simulink model "EGRVlv_VDSens"  (R2016b)
settings: configuration reference "CodeGenConfigSet" (kept outside this file)
values from neighbouring files (symbols this model uses):
  EGRVlv_facAdapClsStrt_C = Calibration.Parameter    [init_EGRVlv_VDSens.m]
  EGRVlv_facAdapPosCls_C = Calibration.Parameter    [init_EGRVlv_VDSens.m]
  EGRVlv_facPT1_C = Calibration.Parameter    [init_EGRVlv_VDSens.m]
  EGRVlv_facPT1ModVal_C = Calibration.Parameter    [init_EGRVlv_VDSens.m]
  EGRVlv_IKiOfsLrnUp_C = Calibration.Parameter    [init_EGRVlv_VDSens.m]
  EGRVlv_numAdapClsMax_C = Calibration.Parameter    [init_EGRVlv_VDSens.m]
  EGRVlv_numEngTempOfsLrnRls1_C = Calibration.Parameter    [init_EGRVlv_VDSens.m]
  EGRVlv_numEngTempOfsLrnRls2_C = Calibration.Parameter    [init_EGRVlv_VDSens.m]
  EGRVlv_numTempSel_C = Calibration.Parameter    [init_EGRVlv_VDSens.m]
  EGRVlv_rActMax_C = Calibration.Parameter    [init_EGRVlv_VDSens.m]
  EGRVlv_rActMin_C = Calibration.Parameter    [init_EGRVlv_VDSens.m]
  EGRVlv_rActOfs_C = Calibration.Parameter    [init_EGRVlv_VDSens.m]
  EGRVlv_rAdapAgOpnMax_C = Calibration.Parameter    [init_EGRVlv_VDSens.m]
  EGRVlv_rAdapAgOpnMin_C = Calibration.Parameter    [init_EGRVlv_VDSens.m]
  EGRVlv_rAdapDiffPlaus_C = Calibration.Parameter    [init_EGRVlv_VDSens.m]
  EGRVlv_rAdapDiffPlausLgT_C = Calibration.Parameter    [init_EGRVlv_VDSens.m]
  EGRVlv_rAdapDiffPlausShT_C = Calibration.Parameter    [init_EGRVlv_VDSens.m]
  EGRVlv_rAdapIniOpn0_C = Calibration.Parameter    [init_EGRVlv_VDSens.m]
  EGRVlv_rAdapIniOpn_C = Calibration.Parameter    [init_EGRVlv_VDSens.m]
  EGRVlv_rAdapOpnBnd_C = Calibration.Parameter    [init_EGRVlv_VDSens.m]
  EGRVlv_rCmpNewCtlUn_C = Calibration.Parameter    [init_EGRVlv_VDSens.m]
  EGRVlv_RmpSlpNeg_C = Calibration.Parameter    [init_EGRVlv_VDSens.m]
  EGRVlv_RmpSlpPos_C = Calibration.Parameter    [init_EGRVlv_VDSens.m]
  EGRVlv_rOfsLrnDwn_C = Calibration.Parameter    [init_EGRVlv_VDSens.m]
  EGRVlv_rOfsLrnRmpDwnCls_C = Calibration.Parameter    [init_EGRVlv_VDSens.m]
  EGRVlv_rOfsLrnRmpUpFst_C = Calibration.Parameter    [init_EGRVlv_VDSens.m]
  EGRVlv_rOfsLrnVlvMax_C = Calibration.Parameter    [init_EGRVlv_VDSens.m]
  EGRVlv_rOfsLrnVlvMin_C = Calibration.Parameter    [init_EGRVlv_VDSens.m]
  EGRVlv_rOfsMax_C = Calibration.Parameter    [init_EGRVlv_VDSens.m]
  EGRVlv_rOfsMin_C = Calibration.Parameter    [init_EGRVlv_VDSens.m]
  EGRVlv_rPullDwnThres_C = Calibration.Parameter    [init_EGRVlv_VDSens.m]
  EGRVlv_rRmpDwnCls_C = Calibration.Parameter    [init_EGRVlv_VDSens.m]
  EGRVlv_rRmpUpFst_C = Calibration.Parameter    [init_EGRVlv_VDSens.m]
  EGRVlv_rSensVlvThres_C = Calibration.Parameter    [init_EGRVlv_VDSens.m]
  EGRVlv_rTmpOfsLrnMax_C = Calibration.Parameter    [init_EGRVlv_VDSens.m]
  EGRVlv_rTmpOfsLrnMin_C = Calibration.Parameter    [init_EGRVlv_VDSens.m]
  EGRVlv_rTransStgDfl_C = Calibration.Parameter    [init_EGRVlv_VDSens.m]
  EGRVlv_stNewVlvTrg_C = Calibration.Parameter    [init_EGRVlv_VDSens.m]
  EGRVlv_stOfsEngCond_C = Calibration.Parameter    [init_EGRVlv_VDSens.m]
  EGRVlv_stOfsLrnEnb_C = Calibration.Parameter    [init_EGRVlv_VDSens.m]
  EGRVlv_stOfsLrnTrg_C = Calibration.Parameter    [init_EGRVlv_VDSens.m]
  EGRVlv_swtActOfs_C = Calibration.Parameter    [init_EGRVlv_VDSens.m]
  EGRVlv_swtOfsLrnActv_C = Calibration.Parameter    [init_EGRVlv_VDSens.m]
  EGRVlv_swtSensPrs_C = Calibration.Parameter    [init_EGRVlv_VDSens.m]
  EGRVlv_tEngFldThresOfsLrnRls1_C = Calibration.Parameter    [init_EGRVlv_VDSens.m]
  EGRVlv_tEngFldThresOfsLrnRls2_C = Calibration.Parameter    [init_EGRVlv_VDSens.m]
  EGRVlv_tEngMax_C = Calibration.Parameter    [init_EGRVlv_VDSens.m]
  EGRVlv_tEngMin_C = Calibration.Parameter    [init_EGRVlv_VDSens.m]
  EGRVlv_tiAdapJamVlv_C = Calibration.Parameter    [init_EGRVlv_VDSens.m]
  EGRVlv_tiAdapWaitSensAcq_C = Calibration.Parameter    [init_EGRVlv_VDSens.m]
  EGRVlv_tiClsJamVlv_C = Calibration.Parameter    [init_EGRVlv_VDSens.m]
  EGRVlv_tiStable_C = Calibration.Parameter    [init_EGRVlv_VDSens.m]
  EGRVlv_uBattMax_C = Calibration.Parameter    [init_EGRVlv_VDSens.m]
  EGRVlv_uBattMin_C = Calibration.Parameter    [init_EGRVlv_VDSens.m]
  PRC_ZERO = fi(0,Prc_100_rate)    [init_EGRVlv_VDSens.m]
  SigTst_rEGRVlv_C = Calibration.Parameter    [init_EGRVlv_VDSens.m]
  SigTst_swtEGRVlv_C = Calibration.Parameter    [init_EGRVlv_VDSens.m]
undefined symbols (not defined in the file or in its folder): CEngDst_switch_conv, EGRVlv_VDSens_DT, EngState_conv, SubSysExeState_conv, Switch_conv
libraries: simulink x22, CXLib x18
(part 2 of 2)

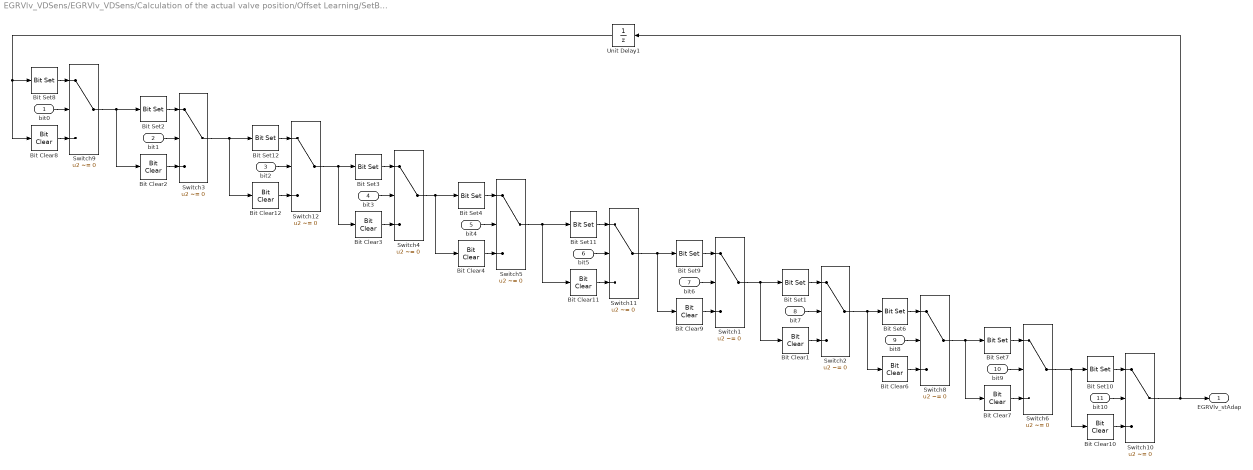
== system EGRVlv_VDSens/EGRVlv_VDSens/Calculation of the actual valve position/Offset Learning/SetBit ==
  bit0 : Inport
  bit1 : Inport  Port=2
  bit2 : Inport  Port=3
  bit3 : Inport  Port=4
  bit4 : Inport  Port=5
  bit5 : Inport  Port=6
  bit6 : Inport  Port=7
  bit7 : Inport  Port=8
  bit8 : Inport  Port=9
  bit9 : Inport  Port=10
  bit10 : Inport  Port=11
  Bit Clear1 : simulink/Logic and Bit Operations/Bit Clear  iBit=7
  Bit Clear10 : simulink/Logic and Bit Operations/Bit Clear  iBit=10
  Bit Clear11 : simulink/Logic and Bit Operations/Bit Clear  iBit=5
  Bit Clear12 : simulink/Logic and Bit Operations/Bit Clear  iBit=2
  Bit Clear2 : simulink/Logic and Bit Operations/Bit Clear  iBit=1
  Bit Clear3 : simulink/Logic and Bit Operations/Bit Clear  iBit=3
  Bit Clear4 : simulink/Logic and Bit Operations/Bit Clear  iBit=4
  Bit Clear6 : simulink/Logic and Bit Operations/Bit Clear  iBit=8
  Bit Clear7 : simulink/Logic and Bit Operations/Bit Clear  iBit=9
  Bit Clear8 : simulink/Logic and Bit Operations/Bit Clear  iBit=0
  Bit Clear9 : simulink/Logic and Bit Operations/Bit Clear  iBit=6
  Bit Set1 : simulink/Logic and Bit Operations/Bit Set  iBit=7
  Bit Set10 : simulink/Logic and Bit Operations/Bit Set  iBit=10
  Bit Set11 : simulink/Logic and Bit Operations/Bit Set  iBit=5
  Bit Set12 : simulink/Logic and Bit Operations/Bit Set  iBit=2
  Bit Set2 : simulink/Logic and Bit Operations/Bit Set  iBit=1
  Bit Set3 : simulink/Logic and Bit Operations/Bit Set  iBit=3
  Bit Set4 : simulink/Logic and Bit Operations/Bit Set  iBit=4
  Bit Set6 : simulink/Logic and Bit Operations/Bit Set  iBit=8
  Bit Set7 : simulink/Logic and Bit Operations/Bit Set  iBit=9
  Bit Set8 : simulink/Logic and Bit Operations/Bit Set  iBit=0
  Bit Set9 : simulink/Logic and Bit Operations/Bit Set  iBit=6
  Switch{1..6,8..12} (11 alike) : Switch  Criteria=u2 ~= 0  OutDataTypeStr=Inherit: Inherit via back propagation  SaturateOnIntegerOverflow=on  InputSameDT=on
  Unit Delay1 : UnitDelay  SampleTime=-1
      settings: AttributesFormatString=InitialValue=%<InitialCondition>
  EGRVlv_stAdap : Outport
  wires:
  bit6/1 -> Switch1/2
  Bit Clear9/1 -> Switch1/3
  bit7/1 -> Switch2/2
  Bit Set9/1 -> Switch1/1
  Switch10/1 -> EGRVlv_stAdap/1, Unit Delay1/1
  Bit Set1/1 -> Switch2/1
  Switch1/1 -> Bit Clear1/1, Bit Set1/1
  Bit Clear1/1 -> Switch2/3
  Bit Clear2/1 -> Switch3/3
  Bit Set2/1 -> Switch3/1
  Bit Clear3/1 -> Switch4/3
  Bit Set3/1 -> Switch4/1
  Unit Delay1/1 -> Bit Clear8/1, Bit Set8/1
  Bit Clear4/1 -> Switch5/3
  Bit Set4/1 -> Switch5/1
  Switch4/1 -> Bit Set4/1, Bit Clear4/1
  bit9/1 -> Switch6/2
  Bit Clear7/1 -> Switch6/3
  Bit Set7/1 -> Switch6/1
  bit8/1 -> Switch8/2
  Bit Clear6/1 -> Switch8/3
  Bit Set6/1 -> Switch8/1
  Switch8/1 -> Bit Set7/1, Bit Clear7/1
  Switch2/1 -> Bit Set6/1, Bit Clear6/1
  Bit Clear8/1 -> Switch9/3
  Bit Set8/1 -> Switch9/1
  Switch9/1 -> Bit Set2/1, Bit Clear2/1
  bit10/1 -> Switch10/2
  Bit Set10/1 -> Switch10/1
  Bit Clear10/1 -> Switch10/3
  Switch6/1 -> Bit Clear10/1, Bit Set10/1
  Bit Clear11/1 -> Switch11/3
  Bit Set11/1 -> Switch11/1
  Switch5/1 -> Bit Clear11/1, Bit Set11/1
  Switch11/1 -> Bit Clear9/1, Bit Set9/1
  bit0/1 -> Switch9/2
  bit1/1 -> Switch3/2
  bit3/1 -> Switch4/2
  bit4/1 -> Switch5/2
  bit5/1 -> Switch11/2
  Bit Clear12/1 -> Switch12/3
  Bit Set12/1 -> Switch12/1
  bit2/1 -> Switch12/2
  Switch12/1 -> Bit Clear3/1, Bit Set3/1
  Switch3/1 -> Bit Clear12/1, Bit Set12/1

== system EGRVlv_VDSens/EGRVlv_VDSens/Calculation of the actual valve position/Offset Learning/State INIT ==
  function : TriggerPort  TriggerType=function-call  VariantControl=Variant
  Constant{,1..3} (4 alike) : Constant  Value=0  OutDataTypeStr=Prc_100_rate
  Constant4 : Constant  Value=0  OutDataTypeStr=Counter_num
  EGRVlv_rAdapLrn_mp : Outport  Tag=%  InitialOutput=0
  EGRVlv_rPosLrnMax_mp : Outport  Tag=%  Port=2
  EGRVlv_rPosLrnMin_mp : Outport  Tag=%  Port=3
  EGRVlv_rAdapPosAvg_mp : Outport  Tag=%  Port=4
  EGRVlv_ctAdapCls_mp : Outport  Port=5
  wires:
  Constant/1 -> EGRVlv_rAdapLrn_mp/1
  Constant1/1 -> EGRVlv_rPosLrnMax_mp/1
  Constant3/1 -> EGRVlv_rAdapPosAvg_mp/1
  Constant2/1 -> EGRVlv_rPosLrnMin_mp/1
  Constant4/1 -> EGRVlv_ctAdapCls_mp/1

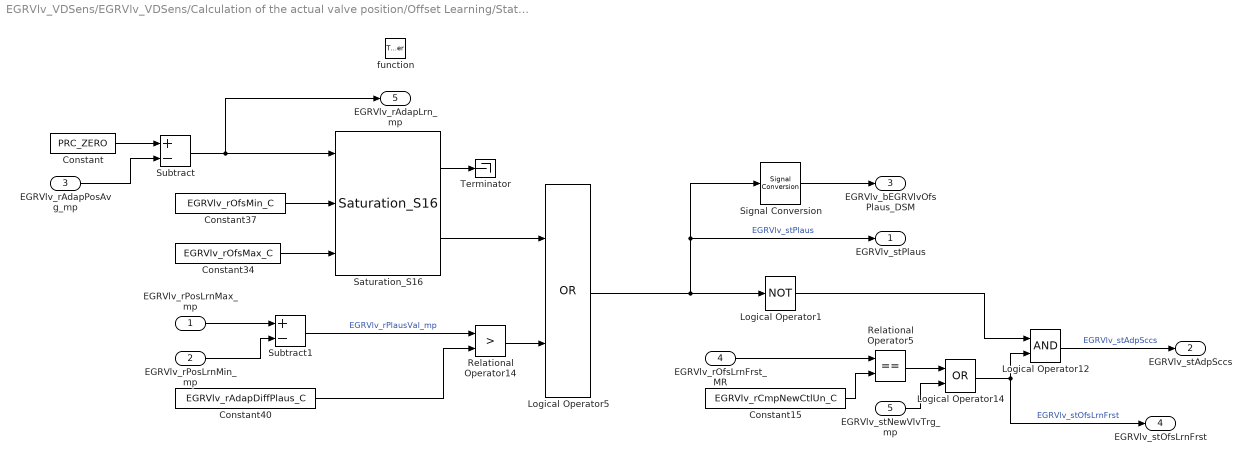
== system EGRVlv_VDSens/EGRVlv_VDSens/Calculation of the actual valve position/Offset Learning/State PLAUSIBLE ==
  EGRVlv_rPosLrnMax_mp : Inport  Tag=%
  EGRVlv_rPosLrnMin_mp : Inport  Tag=%  Port=2
  EGRVlv_rAdapPosAvg_mp : Inport  Tag=%  Port=3
  EGRVlv_rOfsLrnFrst_MR : Inport  Tag=%  Port=4
  EGRVlv_stNewVlvTrg_mp : Inport  Tag=%  Port=5
  function : TriggerPort  TriggerType=function-call  VariantControl=Variant
  Constant : Constant  Value=PRC_ZERO
  Constant15 : Constant  Value=EGRVlv_rCmpNewCtlUn_C  SampleTime=-1
  Constant34 : Constant  Value=EGRVlv_rOfsMax_C  SampleTime=-1
  Constant37 : Constant  Value=EGRVlv_rOfsMin_C  SampleTime=-1
  Constant40 : Constant  Value=EGRVlv_rAdapDiffPlaus_C  SampleTime=-1
  Logical Operator1 : Logic  Operator=NOT  AllPortsSameDT=off  OutDataTypeStr=boolean
  Logical Operator12 : Logic  AllPortsSameDT=off  OutDataTypeStr=boolean
  Logical Operator14 : Logic  Operator=OR  AllPortsSameDT=off  OutDataTypeStr=boolean
  Logical Operator5 : Logic  Operator=OR  AllPortsSameDT=off  OutDataTypeStr=boolean
  Relational Operator14 : RelationalOperator  Operator=>  OutDataTypeStr=boolean  RndMeth=Simplest
  Relational Operator5 : RelationalOperator  Operator===  OutDataTypeStr=boolean  RndMeth=Simplest
  Saturation_S16 : CXLib/Saturation_S16
  Signal Conversion : SignalConversion  OverrideOpt=off
  Subtract : Sum  Inputs=+-  OutDataTypeStr=Inherit: Inherit via back propagation  SaturateOnIntegerOverflow=on  InputSameDT=on
  Subtract1 : Sum  Inputs=+-  SaturateOnIntegerOverflow=on
  Terminator : Terminator
  EGRVlv_stPlaus : Outport  Tag=%
  EGRVlv_stAdpSccs : Outport  Tag=%  Port=2
  EGRVlv_bEGRVlvOfsPlaus_DSM : Outport  Tag=%  Port=3
  EGRVlv_stOfsLrnFrst : Outport  Port=4
  EGRVlv_rAdapLrn_mp : Outport  Tag=%  Port=5  InitialOutput=0
  wires:
  Logical Operator5/1 -> EGRVlv_stPlaus/1, Signal Conversion/1, Logical Operator1/1  "EGRVlv_stPlaus"
  Saturation_S16/2 -> Logical Operator5/1
  Relational Operator14/1 -> Logical Operator5/2
  Subtract1/1 -> Relational Operator14/1  "EGRVlv_rPlausVal_mp"
  Constant40/1 -> Relational Operator14/2
  Constant37/1 -> Saturation_S16/2
  Constant34/1 -> Saturation_S16/3
  Subtract/1 -> Saturation_S16/1, EGRVlv_rAdapLrn_mp/1
  EGRVlv_rPosLrnMax_mp/1 -> Subtract1/1
  EGRVlv_rPosLrnMin_mp/1 -> Subtract1/2
  Signal Conversion/1 -> EGRVlv_bEGRVlvOfsPlaus_DSM/1
  Constant/1 -> Subtract/1
  Logical Operator1/1 -> Logical Operator12/1
  EGRVlv_rOfsLrnFrst_MR/1 -> Relational Operator5/1
  Constant15/1 -> Relational Operator5/2
  Relational Operator5/1 -> Logical Operator14/1
  EGRVlv_stNewVlvTrg_mp/1 -> Logical Operator14/2
  Logical Operator14/1 -> EGRVlv_stOfsLrnFrst/1, Logical Operator12/2  "EGRVlv_stOfsLrnFrst"
  Logical Operator12/1 -> EGRVlv_stAdpSccs/1  "EGRVlv_stAdpSccs"
  EGRVlv_rAdapPosAvg_mp/1 -> Subtract/2
  Saturation_S16/1 -> Terminator/1

== system EGRVlv_VDSens/EGRVlv_VDSens/Calculation of the actual valve position/Offset Learning/State machine for the offset learning for EGR valve/simfcn ==
  EGRVlv_rOfsLrnVlv : Inport  Tag=%
  EGRVlv_rActUnCor : Inport  Port=2  OutDataTypeStr=Prc_100_rate
  EGRVlv_rOfsLrnLst_MR : Inport  Port=3  OutDataTypeStr=Prc_100_rate
  f : TriggerPort  TriggerType=function-call  VariantControl=Variant
      settings: CopyFcn=Stateflow.SLINSF.SimulinkMan.removeBlockPreDeleteFcn  PreDeleteFcn=Stateflow.SLINSF.SimulinkMan.unsafePredeleteFcn
  Add1 : Sum  OutDataTypeStr=Prc_100_rate  SaturateOnIntegerOverflow=on
  Constant10 : Constant  OutDataTypeStr=Prc_100_rate
  Constant11 : Constant  Value=EGRVlv_rAdapOpnBnd_C
  Constant13 : Constant  Value=EGRVlv_rAdapAgOpnMax_C
  Constant7 : Constant  Value=EGRVlv_IKiOfsLrnUp_C
  Integral : Subsystem
  Relational Operator2 : RelationalOperator  OutDataTypeStr=boolean  RndMeth=Simplest
  Switch : Switch  Criteria=u2 ~= 0
  EGRVlv_rOfsLrnVlvUnLim : Outport
  wires:
  Constant10/1 -> Integral/1(Dvt)
  Add1/1 -> Relational Operator2/1
  Constant13/1 -> Relational Operator2/2
  EGRVlv_rActUnCor/1 -> Add1/1
  EGRVlv_rOfsLrnLst_MR/1 -> Add1/2
  Relational Operator2/1 -> Switch/2
  Constant11/1 -> Switch/1
  Switch/1 -> EGRVlv_rOfsLrnVlvUnLim/1
  Integral/1(Out) -> Switch/3
  EGRVlv_rOfsLrnVlv/1 -> Integral/3(InitVal)
  Constant7/1 -> Integral/2(Ki)

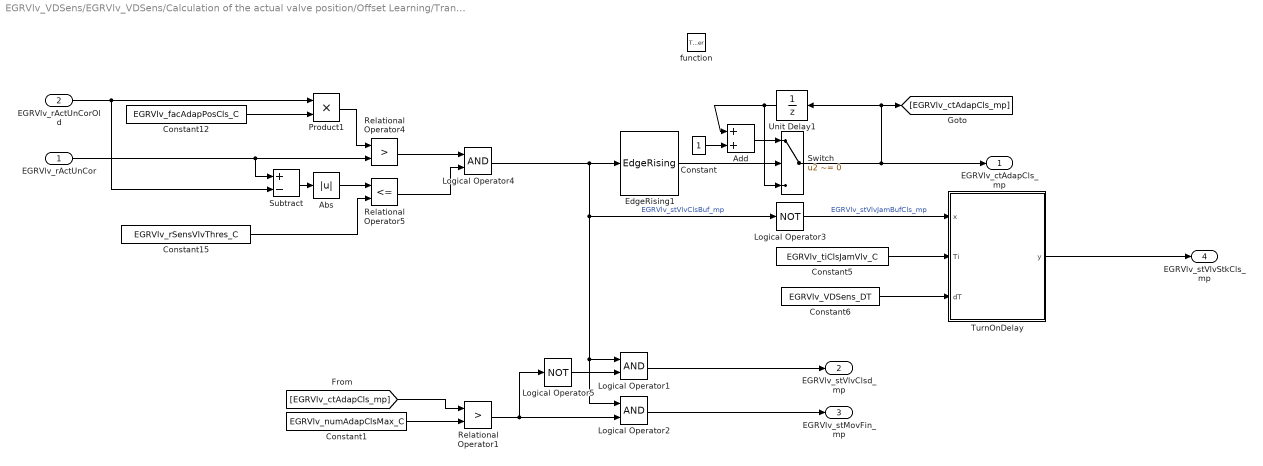
== system EGRVlv_VDSens/EGRVlv_VDSens/Calculation of the actual valve position/Offset Learning/Transition conditions from state CLOSE ==
  EGRVlv_rActUnCor : Inport
  EGRVlv_rActUnCorOld : Inport  Port=2
  function : TriggerPort  TriggerType=function-call  VariantControl=Variant  StatesWhenEnabling=reset
  Abs : Abs
  Add : Sum  SaturateOnIntegerOverflow=on
  Constant : Constant  OutDataTypeStr=Counter_num
  Constant1 : Constant  Value=EGRVlv_numAdapClsMax_C
  Constant12 : Constant  Value=EGRVlv_facAdapPosCls_C
  Constant15 : Constant  Value=EGRVlv_rSensVlvThres_C
  Constant5 : Constant  Value=EGRVlv_tiClsJamVlv_C
  Constant6 : Constant  Value=EGRVlv_VDSens_DT
  EdgeRising1 : CXLib/EdgeRising
  Logical Operator1 : Logic  AllPortsSameDT=off  OutDataTypeStr=boolean
  Logical Operator2 : Logic  AllPortsSameDT=off  OutDataTypeStr=boolean
  Logical Operator3 : Logic  Operator=NOT  AllPortsSameDT=off  OutDataTypeStr=boolean
  Logical Operator4 : Logic  AllPortsSameDT=off  OutDataTypeStr=boolean
  Logical Operator5 : Logic  Operator=NOT  AllPortsSameDT=off  OutDataTypeStr=boolean
  Product1 : Product  OutDataTypeStr=Prc_100_rate  SaturateOnIntegerOverflow=on
  Relational Operator1 : RelationalOperator  Operator=>  OutDataTypeStr=boolean  RndMeth=Simplest
  Relational Operator4 : RelationalOperator  Operator=>  OutDataTypeStr=boolean  RndMeth=Simplest
  Relational Operator5 : RelationalOperator  Operator=<=  OutDataTypeStr=boolean  RndMeth=Simplest
  Subtract : Sum  Inputs=+-  SaturateOnIntegerOverflow=on
  Switch : Switch  Criteria=u2 ~= 0
  TurnOnDelay : Subsystem
  Unit Delay1 : UnitDelay  SampleTime=-1
      settings: AttributesFormatString=InitialValue=%<InitialCondition>
  EGRVlv_ctAdapCls_mp : Outport
  EGRVlv_stVlvClsd_mp : Outport  Port=2  InitialOutput=0
  EGRVlv_stMovFin_mp : Outport  Port=3  InitialOutput=0
  EGRVlv_stVlvStkCls_mp : Outport  Port=4  InitialOutput=0
  wires:
  Logical Operator4/1 -> EdgeRising1/1, Logical Operator3/1, Logical Operator2/1, Logical Operator1/1  "EGRVlv_stVlvClsBuf_mp"
  Constant5/1 -> TurnOnDelay/2(Ti)
  Constant6/1 -> TurnOnDelay/3(dT)
  Logical Operator3/1 -> TurnOnDelay/1(x)  "EGRVlv_stVlvJamBufCls_mp"
  EGRVlv_rActUnCor/1 -> Subtract/1, Relational Operator4/2
  Constant12/1 -> Product1/2
  Product1/1 -> Relational Operator4/1
  Relational Operator4/1 -> Logical Operator4/1
  EGRVlv_rActUnCorOld/1 -> Subtract/2, Product1/1
  Subtract/1 -> Abs/1
  Abs/1 -> Relational Operator5/1
  Constant15/1 -> Relational Operator5/2
  Relational Operator5/1 -> Logical Operator4/2
  Constant/1 -> Add/2
  Add/1 -> Switch/1
  Unit Delay1/1 -> Switch/3, Add/1
  Switch/1 -> EGRVlv_ctAdapCls_mp/1, Unit Delay1/1, [EGRVlv_ctAdapCls_mp]
  Logical Operator1/1 -> EGRVlv_stVlvClsd_mp/1
  Logical Operator2/1 -> EGRVlv_stMovFin_mp/1
  Logical Operator5/1 -> Logical Operator1/2
  Constant1/1 -> Relational Operator1/2
  Relational Operator1/1 -> Logical Operator5/1, Logical Operator2/2
  [EGRVlv_ctAdapCls_mp] -> Relational Operator1/1
  EdgeRising1/1 -> Switch/2
  TurnOnDelay/1(y) -> EGRVlv_stVlvStkCls_mp/1

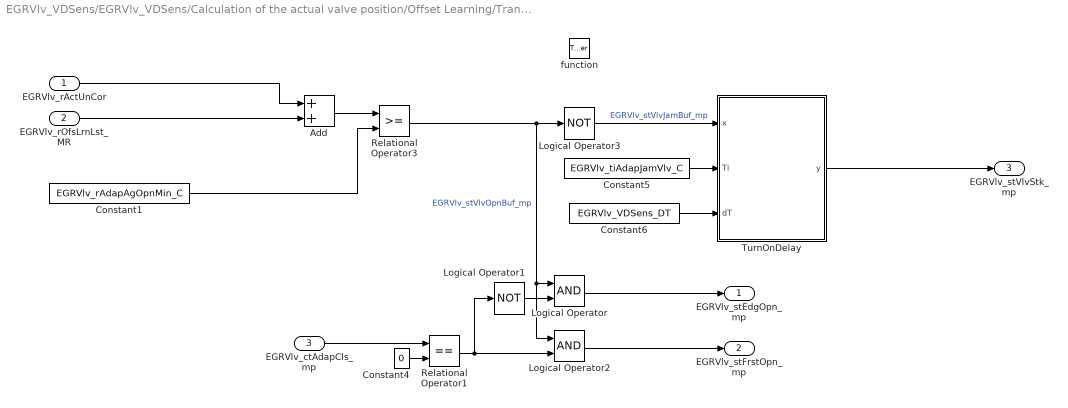
== system EGRVlv_VDSens/EGRVlv_VDSens/Calculation of the actual valve position/Offset Learning/Transition conditions from state OPEN ==
  EGRVlv_rActUnCor : Inport
  EGRVlv_rOfsLrnLst_MR : Inport  Port=2
  EGRVlv_ctAdapCls_mp : Inport  Tag=%  Port=3
  function : TriggerPort  TriggerType=function-call  VariantControl=Variant
  Add : Sum  SaturateOnIntegerOverflow=on
  Constant1 : Constant  Value=EGRVlv_rAdapAgOpnMin_C
  Constant4 : Constant  Value=0  OutDataTypeStr=Inherit: Inherit via back propagation
  Constant5 : Constant  Value=EGRVlv_tiAdapJamVlv_C
  Constant6 : Constant  Value=EGRVlv_VDSens_DT
  Logical Operator : Logic  AllPortsSameDT=off  OutDataTypeStr=boolean
  Logical Operator1 : Logic  Operator=NOT  AllPortsSameDT=off  OutDataTypeStr=boolean
  Logical Operator2 : Logic  AllPortsSameDT=off  OutDataTypeStr=boolean
  Logical Operator3 : Logic  Operator=NOT  AllPortsSameDT=off  OutDataTypeStr=boolean
  Relational Operator1 : RelationalOperator  Operator===  OutDataTypeStr=boolean  RndMeth=Simplest  InputSameDT=on
  Relational Operator3 : RelationalOperator  OutDataTypeStr=boolean  RndMeth=Simplest
  TurnOnDelay : Subsystem
  EGRVlv_stEdgOpn_mp : Outport  InitialOutput=0
  EGRVlv_stFrstOpn_mp : Outport  Port=2  InitialOutput=0
  EGRVlv_stVlvStk_mp : Outport  Port=3  InitialOutput=0
  wires:
  Add/1 -> Relational Operator3/1
  Constant1/1 -> Relational Operator3/2
  Relational Operator3/1 -> Logical Operator2/1, Logical Operator/1, Logical Operator3/1  "EGRVlv_stVlvOpnBuf_mp"
  EGRVlv_ctAdapCls_mp/1 -> Relational Operator1/1
  Constant4/1 -> Relational Operator1/2
  Logical Operator1/1 -> Logical Operator/2
  Relational Operator1/1 -> Logical Operator1/1, Logical Operator2/2
  Logical Operator/1 -> EGRVlv_stEdgOpn_mp/1
  Logical Operator2/1 -> EGRVlv_stFrstOpn_mp/1
  Constant5/1 -> TurnOnDelay/2(Ti)
  Constant6/1 -> TurnOnDelay/3(dT)
  Logical Operator3/1 -> TurnOnDelay/1(x)  "EGRVlv_stVlvJamBuf_mp"
  EGRVlv_rOfsLrnLst_MR/1 -> Add/2
  EGRVlv_rActUnCor/1 -> Add/1
  TurnOnDelay/1(y) -> EGRVlv_stVlvStk_mp/1

== system EGRVlv_VDSens/EGRVlv_VDSens/Calculation of the actual valve position/Offset Learning/Transition conditions from state Store ==
  EGRVlv_rAdapPos_mp : Inport  Tag=%
  EGRVlv_ctAdapCls_mp : Inport  Tag=%  Port=2
  function : TriggerPort  TriggerType=function-call  VariantControl=Variant
  Add : Sum  SaturateOnIntegerOverflow=on
  Constant1 : Constant  Value=0  OutDataTypeStr=Counter_num  SampleTime=-1
  Divide : Product  Inputs=*/  OutDataTypeStr=Prc_100_rate  SaturateOnIntegerOverflow=on
  Relational Operator1 : RelationalOperator  Operator=~=  OutDataTypeStr=boolean  RndMeth=Simplest
  Relational Operator4 : RelationalOperator  Operator=>  OutDataTypeStr=boolean  RndMeth=Simplest
  Relational Operator5 : RelationalOperator  Operator=<  OutDataTypeStr=boolean  RndMeth=Simplest
  Switch1 : Switch  Criteria=u2 ~= 0  Threshold=CEngDst_switch_conv.OFF  InputSameDT=on
  Switch7 : Switch  Criteria=u2 ~= 0  Threshold=CEngDst_switch_conv.OFF  InputSameDT=on
  Switch8 : Switch  Criteria=u2 ~= 0  Threshold=CEngDst_switch_conv.OFF  InputSameDT=on
  Unit Delay : UnitDelay  InitialCondition=-100  SampleTime=-1
      settings: AttributesFormatString=InitialValue=%<InitialCondition>
  Unit Delay1 : UnitDelay  InitialCondition=100  SampleTime=-1
      settings: AttributesFormatString=InitialValue=%<InitialCondition>
  Unit Delay2 : UnitDelay  SampleTime=-1
      settings: AttributesFormatString=InitialValue=%<InitialCondition>
  EGRVlv_rPosLrnMax_mp : Outport  Tag=%
  EGRVlv_rPosLrnMin_mp : Outport  Tag=%  Port=2
  EGRVlv_rAdapPosAvg_mp : Outport  Tag=%  Port=3
  wires:
  Relational Operator1/1 -> Switch1/2
  Unit Delay/1 -> Relational Operator4/2, Switch7/3
  Unit Delay1/1 -> Switch8/3, Relational Operator5/2
  Switch8/1 -> EGRVlv_rPosLrnMin_mp/1, Unit Delay1/1
  Relational Operator5/1 -> Switch8/2
  Relational Operator4/1 -> Switch7/2
  Constant1/1 -> Relational Operator1/2
  Divide/1 -> Switch1/1
  Unit Delay2/1 -> Add/1
  EGRVlv_ctAdapCls_mp/1 -> Relational Operator1/1, Divide/2
  Switch7/1 -> EGRVlv_rPosLrnMax_mp/1, Unit Delay/1
  EGRVlv_rAdapPos_mp/1 -> Switch1/3, Switch8/1, Relational Operator5/1, Relational Operator4/1, Switch7/1, Add/2
  Switch1/1 -> EGRVlv_rAdapPosAvg_mp/1
  Add/1 -> Divide/1, Unit Delay2/1

== system EGRVlv_VDSens/EGRVlv_VDSens/Calculation of the actual valve position/Offset Learning/State machine for the offset learning for EGR valve/simfcn/Integral ==
  note: Outport
      | should inherit data type from back
  Dvt : Inport
  Ki : Inport  Port=2
  InitVal : Inport  Port=3
  Data Type Duplicate : DataTypeDuplicate
  Product3 : Product  OutDataTypeStr=Inherit: Inherit via back propagation  SaturateOnIntegerOverflow=on
  Sum : Sum  OutDataTypeStr=Inherit: Inherit via back propagation  SaturateOnIntegerOverflow=on  InputSameDT=on
  Out : Outport
  wires:
  Dvt/1 -> Product3/1
  Sum/1 -> Out/1, Data Type Duplicate/1
  InitVal/1 -> Sum/1, Data Type Duplicate/2
  Product3/1 -> Sum/2
  Ki/1 -> Product3/2

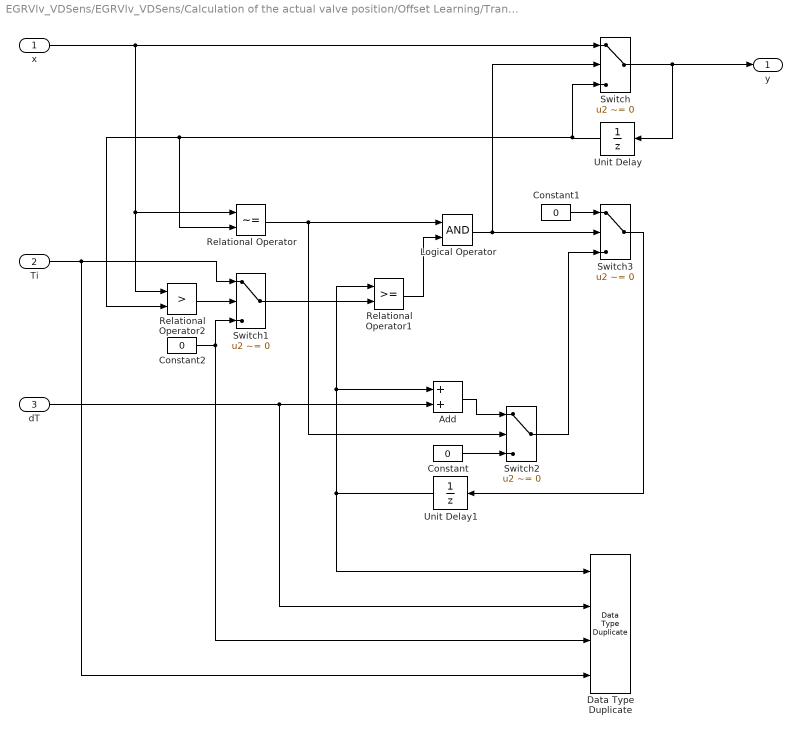
== system EGRVlv_VDSens/EGRVlv_VDSens/Calculation of the actual valve position/Offset Learning/Transition conditions from state CLOSE/TurnOnDelay ==
  x : Inport
  Ti : Inport  Port=2
  dT : Inport  Port=3
  Add : Sum  SaturateOnIntegerOverflow=on
  Constant : Constant  Value=0  OutDataTypeStr=Inherit: Inherit via back propagation
  Constant1 : Constant  Value=0  OutDataTypeStr=Inherit: Inherit via back propagation
  Constant2 : Constant  Value=0  OutDataTypeStr=Inherit: Inherit via back propagation
  Data Type Duplicate : DataTypeDuplicate  NumInputPorts=4
  Logical Operator : Logic  OutDataTypeStr=boolean
  Relational Operator : RelationalOperator  Operator=~=  OutDataTypeStr=boolean  RndMeth=Simplest  InputSameDT=on
  Relational Operator1 : RelationalOperator  OutDataTypeStr=boolean  RndMeth=Simplest  InputSameDT=on
  Relational Operator2 : RelationalOperator  Operator=>  OutDataTypeStr=boolean  RndMeth=Simplest  InputSameDT=on
  Switch{,1..3} (4 alike) : Switch  Criteria=u2 ~= 0  InputSameDT=on
  Unit Delay : UnitDelay  SampleTime=-1
  Unit Delay1 : UnitDelay  SampleTime=-1
  y : Outport
  wires:
  Relational Operator/1 -> Logical Operator/1, Switch2/2
  dT/1 -> Data Type Duplicate/2, Add/2
  Unit Delay1/1 -> Relational Operator1/1, Add/1, Data Type Duplicate/1
  Constant2/1 -> Data Type Duplicate/3, Switch1/3
  x/1 -> Switch/1, Relational Operator2/1, Relational Operator/1
  Switch2/1 -> Switch3/3
  Constant1/1 -> Switch3/1
  Unit Delay/1 -> Relational Operator2/2, Relational Operator/2, Switch/3
  Relational Operator2/1 -> Switch1/2
  Switch3/1 -> Unit Delay1/1
  Ti/1 -> Data Type Duplicate/4, Switch1/1
  Constant/1 -> Switch2/3
  Relational Operator1/1 -> Logical Operator/2
  Add/1 -> Switch2/1
  Switch/1 -> y/1, Unit Delay/1
  Switch1/1 -> Relational Operator1/2
  Logical Operator/1 -> Switch/2, Switch3/2

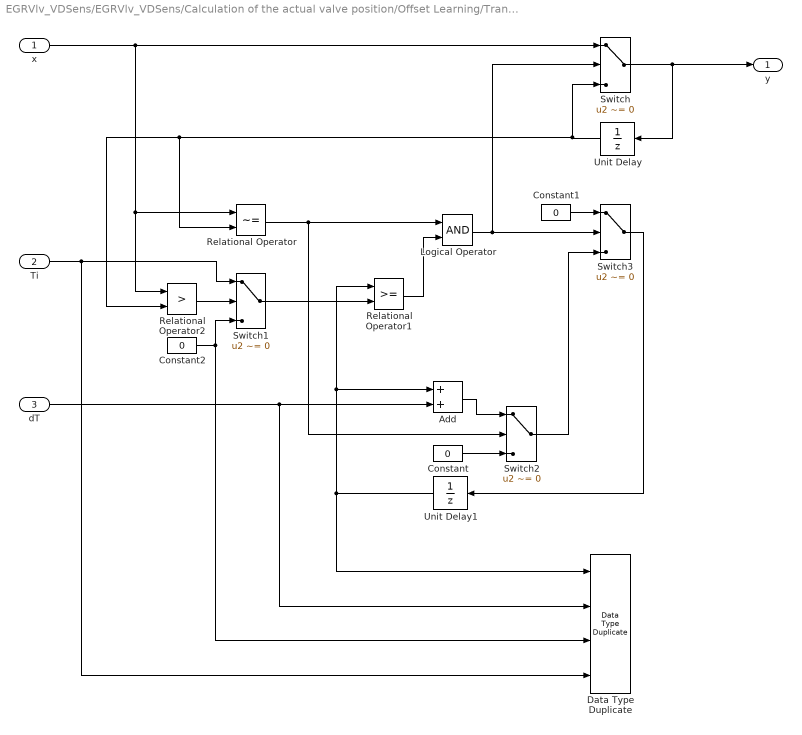
== system EGRVlv_VDSens/EGRVlv_VDSens/Calculation of the actual valve position/Offset Learning/Transition conditions from state OPEN/TurnOnDelay ==
  x : Inport
  Ti : Inport  Port=2
  dT : Inport  Port=3
  Add : Sum  SaturateOnIntegerOverflow=on
  Constant : Constant  Value=0  OutDataTypeStr=Inherit: Inherit via back propagation
  Constant1 : Constant  Value=0  OutDataTypeStr=Inherit: Inherit via back propagation
  Constant2 : Constant  Value=0  OutDataTypeStr=Inherit: Inherit via back propagation
  Data Type Duplicate : DataTypeDuplicate  NumInputPorts=4
  Logical Operator : Logic  OutDataTypeStr=boolean
  Relational Operator : RelationalOperator  Operator=~=  OutDataTypeStr=boolean  RndMeth=Simplest  InputSameDT=on
  Relational Operator1 : RelationalOperator  OutDataTypeStr=boolean  RndMeth=Simplest  InputSameDT=on
  Relational Operator2 : RelationalOperator  Operator=>  OutDataTypeStr=boolean  RndMeth=Simplest  InputSameDT=on
  Switch{,1..3} (4 alike) : Switch  Criteria=u2 ~= 0  InputSameDT=on
  Unit Delay : UnitDelay  SampleTime=-1
  Unit Delay1 : UnitDelay  SampleTime=-1
  y : Outport
  wires:
  Relational Operator/1 -> Logical Operator/1, Switch2/2
  dT/1 -> Data Type Duplicate/2, Add/2
  Unit Delay1/1 -> Relational Operator1/1, Add/1, Data Type Duplicate/1
  Constant2/1 -> Data Type Duplicate/3, Switch1/3
  x/1 -> Switch/1, Relational Operator2/1, Relational Operator/1
  Switch2/1 -> Switch3/3
  Constant1/1 -> Switch3/1
  Unit Delay/1 -> Relational Operator2/2, Relational Operator/2, Switch/3
  Relational Operator2/1 -> Switch1/2
  Switch3/1 -> Unit Delay1/1
  Ti/1 -> Data Type Duplicate/4, Switch1/1
  Constant/1 -> Switch2/3
  Relational Operator1/1 -> Logical Operator/2
  Add/1 -> Switch2/1
  Switch/1 -> y/1, Unit Delay/1
  Switch1/1 -> Relational Operator1/2
  Logical Operator/1 -> Switch/2, Switch3/2

== stateflow chart EGRVlv_VDSens/Calculation of the actual valve position/Offset Learning/State machine for the offset learning for EGR valve ==
  state EGRVlv_rOfsLrnVlvUnLim = simfcn(EGRVlv_rOfsLrnVlv,EGRVlv_rActUnCor,EGRVlv_rOfsLrnLst_MR) [function]
  state EGRVLV_ST_OPN
    entry:
    EGRVlv_stOfsLrn = 2;
    EGRVlv_stAdapVlv_mp = 0;
    Open;
    during:
    Open;
    EGRVlv_rOfsLrnVlvUnLim = simfcn(EGRVlv_rOfsLrnVlv,EGRVlv_rActUnCor,EGRVlv_rOfsLrnLst_MR);
    (default) -> (junction 330)
    (junction 330) -> (junction 331) [order 1] : [EGRVlv_ctAdapCls_mp == 0]
    (junction 330) -> (junction 332) [order 2] : {EGRVlv_rOfsLrnVlvUnLim = EGRVlv_rAdapIniOpn_C;}
    (junction 331) -> (junction 333) : {EGRVlv_rOfsLrnVlvUnLim = EGRVlv_rEGR + EGRVlv_rAdapIniOpn0_C;}
    (junction 333) -> (junction 332)
    (junction 332) -> (junction 334)
  state EGRVLV_ST_CLS
    entry:
    EGRVlv_stOfsLrn = 3;
    EGRVlv_stAdapVlv_mp = 1;
    EGRVlv_rOfsLrnVlvUnLim = EGRVlv_rOfsLrnVlv * EGRVlv_facAdapClsStrt_C;
    Close;
    during:
    Close;
    EGRVlv_rOfsLrnVlvUnLim = EGRVlv_rOfsLrnVlv - EGRVlv_rOfsLrnDwn_C;
  state EGRVLV_ST_INIT
    entry:
    EGRVlv_stOfsLrn = 1;
    EGRVlv_bEGRVlvOfsLrnJamVlv_DSM = 0;
    EGRVlv_stLgTDrft = 0;
    EGRVlv_stShTDrft = 0;
    Init;
  state EGRVLV_ST_RMPDWNCLS
    entry:
    EGRVlv_stOfsLrn = 17;
    EGRVlv_stIntegRmpDwnCls_mp = 0;
    EGRVLV_ST_RMPDWNCLS -> (junction 156) [order 1]
    (junction 156) -> (junction 158) [order 1] : [EGRVlv_rOfsLrnVlvUnLim<=EGRVlv_rRmpDwnCls_C]
    (junction 156) -> (junction 161) [order 2] : {EGRVlv_rOfsLrnVlvUnLim = EGRVlv_rOfsLrnVlv - EGRVlv_rOfsLrnRmpDwnCls_C;}
    (junction 158) -> (junction 160) : {EGRVlv_stIntegRmpDwnCls_mp = 1;}
    (junction 160) -> (junction 161)
    (junction 161) -> (junction 165)
  state EGRVLV_ST_RMPUPFST
    entry:
    EGRVlv_stOfsLrn = 18;
    EGRVlv_stIntegRmpUpFst_mp = 0;
    EGRVLV_ST_RMPUPFST -> (junction 174) [order 1]
    (junction 174) -> (junction 175) [order 1] : [EGRVlv_rOfsLrnVlvUnLim>=EGRVlv_rRmpUpFst_C]
    (junction 174) -> (junction 172) [order 2] : {EGRVlv_rOfsLrnVlvUnLim = EGRVlv_rOfsLrnVlv + EGRVlv_rOfsLrnRmpUpFst_C;}
    (junction 175) -> (junction 169) : {EGRVlv_tiStable_mp+=DT;}
    (junction 169) -> (junction 179) [order 1] : [EGRVlv_tiStable_mp>=EGRVlv_tiStable_C]
    (junction 169) -> (junction 178) [order 2]
    (junction 179) -> (junction 180) : {EGRVlv_stIntegRmpUpFst_mp = 1;}
    (junction 178) -> (junction 172)
    (junction 180) -> (junction 178)
    (junction 172) -> (junction 187)
  state EGRVLV_ST_WAITSENSACQ
    entry:
    EGRVlv_stOfsLrn = 19;
    EGRVlv_stWaitElaps = 0;
    EGRVLV_ST_WAITSENSACQ -> (junction 287) [order 1]
    (junction 287) -> (junction 288) [order 1] : [EGRVlv_tiAdapWaitSensAcq_mp>=EGRVlv_tiAdapWaitSensAcq_C]
    (junction 287) -> (junction 290) [order 2] : {EGRVlv_tiAdapWaitSensAcq_mp+=DT;}
    (junction 288) -> (junction 291) : {EGRVlv_stWaitElaps = 1;
        | EGRVlv_tiAdapWaitSensAcq_mp = 0;}
    (junction 291) -> (junction 290)
    (junction 290) -> (junction 289)
  state EGRVLV_ST_STR
    entry:
    EGRVlv_stOfsLrn = 12;
    EGRVlv_stStr_mp = 0;
    during:
    EGRVlv_rAdapPos_mp = EGRVlv_rActUnCor;
    Store;
    EGRVlv_stStr_mp = 1;
  state EGRVLV_ST_SHOFF
    entry:
    EGRVlv_stOfsLrn = 8;
    EGRVlv_rOfsLrnVlvUnLim = 0;
    EGRVlv_bEGRVlvOfsLrnJamVlv_DSM = 1;
  state EGRVLV_ST_PLAUS
    entry:
    EGRVlv_stOfsLrn = 9;
    Plausible;
    during:
    Plausible;
  state EGRVLV_ST_RMTVAL
    entry:
    EGRVlv_stOfsLrn = 7;
    EGRVlv_rOfsLrnVlvUnLim = 0;
    EGRVlv_stAdapFin = 1;
  state EGRVLV_ST_LGTDRFT
    entry:
    EGRVlv_stOfsLrn = 10;
    EGRVlv_stLgTDrft = 0;
    EGRVlv_bEGRVlvLgTDrft_DSM = 0;
    (default) -> (junction 264)
    EGRVLV_ST_LGTDRFT -> (junction 264) [order 1]
    (junction 264) -> (junction 265) [order 1] : [abs(EGRVlv_rAdapPosAvg_mp-EGRVlv_rOfsLrnFrst_MR)>EGRVlv_rAdapDiffPlausLgT_C]
    (junction 265) -> (junction 268) : {EGRVlv_stLgTDrft = 1;
        | EGRVlv_bEGRVlvLgTDrft_DSM = 1;}
    (junction 264) -> (junction 266) [order 2]
    (junction 268) -> (junction 266)
    (junction 266) -> (junction 267)
  state EGRVLV_ST_SHTDRFT
    entry:
    EGRVlv_stOfsLrn = 11;
    EGRVlv_stShTDrft = 0;
    EGRVlv_bEGRVlvShTDrft_DSM = 0;
    (default) -> (junction 276)
    EGRVLV_ST_SHTDRFT -> (junction 276) [order 1]
    (junction 276) -> (junction 280) [order 1] : [abs(EGRVlv_rAdapPosAvg_mp-EGRVlv_rOfsLrnLst_MR)>EGRVlv_rAdapDiffPlausShT_C]
    (junction 276) -> (junction 281) [order 2]
    (junction 280) -> (junction 275) : {EGRVlv_stShTDrft = 1;
        | EGRVlv_bEGRVlvShTDrft_DSM = 1;}
    (junction 275) -> (junction 281)
    (junction 281) -> (junction 277)
  state EGRVLV_ST_ADAPSCCS
    entry:
    EGRVlv_stOfsLrn = 6;
    EGRVlv_rOfsLrnVlvUnLim = 0;
    EGRVlv_stAdapFin = 1;
    EGRVlv_rOfsLrnLst_MW = EGRVlv_rAdapPosAvg_mp;
    (default) -> (junction 253)
    (junction 253) -> (junction 254) [order 1] : [EGRVlv_stOfsLrnFrst == 1]
    (junction 253) -> (junction 257) [order 2]
    (junction 254) -> (junction 256) : {EGRVlv_rOfsLrnFrst_MW = EGRVlv_rAdapPosAvg_mp;}
    (junction 256) -> (junction 257)
    (junction 257) -> (junction 258)
  (default) -> EGRVLV_ST_INIT : {EGRVlv_rOfsLrnFrst_MW = EGRVlv_rOfsLrnFrst_MR;
      | EGRVlv_rOfsLrnLst_MW = EGRVlv_rOfsLrnLst_MR;}
  EGRVLV_ST_CLS -> EGRVLV_ST_PLAUS [order 2] : [EGRVlv_stMovFin_mp == 1]
  EGRVLV_ST_INIT -> EGRVLV_ST_OPN : [EGRVlv_stTrg_mp == 1]
  EGRVLV_ST_OPN -> EGRVLV_ST_CLS [order 2] : [(EGRVlv_stFrstOpn_mp == 1)||...
      | ((EGRVlv_stEdgOpn_mp == 1)&&...
      | (EGRVlv_swtEGRTyp2 == 1))]
  EGRVLV_ST_CLS -> EGRVLV_ST_SHOFF [order 3] : [EGRVlv_stVlvStkCls_mp == 1]
  EGRVLV_ST_STR -> EGRVLV_ST_CLS [order 2] : [(EGRVlv_stAdapVlv_mp == 0) &&...
      | (EGRVlv_stStr_mp == 1)]
  EGRVLV_ST_CLS -> EGRVLV_ST_RMPDWNCLS [order 1] : [(EGRVlv_stVlvClsd_mp == 1)&&...
      | (EGRVlv_swtEGRTyp2T == 1)]
  EGRVLV_ST_ADAPSCCS -> EGRVLV_ST_INIT
  EGRVLV_ST_RMTVAL -> EGRVLV_ST_INIT
  EGRVLV_ST_OPN -> EGRVLV_ST_SHOFF [order 1] : [EGRVlv_stVlvStk_mp == 1]
  EGRVLV_ST_STR -> EGRVLV_ST_OPN [order 1] : [(EGRVlv_stAdapVlv_mp == 1) &&...
      | (EGRVlv_stStr_mp == 1)]
  EGRVLV_ST_RMPDWNCLS -> EGRVLV_ST_RMPUPFST [order 1] : [(EGRVlv_stIntegRmpDwnCls_mp ==1)&&...
      | ((EGRVlv_swtEGRTyp2T == 1))]
  EGRVLV_ST_RMPUPFST -> EGRVLV_ST_WAITSENSACQ [order 1] : [(EGRVlv_stIntegRmpUpFst_mp ==1)&&...
      | (EGRVlv_swtEGRTyp2T == 1)]
      | {EGRVlv_tiStable_mp =0;}
  EGRVLV_ST_WAITSENSACQ -> EGRVLV_ST_STR [order 1] : [EGRVlv_stWaitElaps == 1]
  EGRVLV_ST_SHOFF -> EGRVLV_ST_RMTVAL
  EGRVLV_ST_PLAUS -> EGRVLV_ST_RMTVAL [order 3] : [EGRVlv_stPlaus ==1]
  EGRVLV_ST_PLAUS -> EGRVLV_ST_ADAPSCCS [order 1] : [EGRVlv_stAdpSccs == 1]
  EGRVLV_ST_PLAUS -> EGRVLV_ST_LGTDRFT [order 2] : [EGRVlv_stPlaus == 0]
  EGRVLV_ST_LGTDRFT -> EGRVLV_ST_RMTVAL [order 2] : [EGRVlv_stLgTDrft ==1]
  EGRVLV_ST_SHTDRFT -> EGRVLV_ST_RMTVAL [order 2] : [EGRVlv_stShTDrft ==1]
  EGRVLV_ST_LGTDRFT -> EGRVLV_ST_SHTDRFT [order 1] : [EGRVlv_stLgTDrft  == 0]
  EGRVLV_ST_SHTDRFT -> EGRVLV_ST_ADAPSCCS [order 1] : [EGRVlv_stShTDrft == 0]
  data: EGRVlv_rOfsLrnVlv function_input; EGRVlv_rOfsLrnVlvUnLim function_output; EGRVlv_rActUnCor function_input Prc_100_rate; EGRVlv_rOfsLrnLst_MR function_input Prc_100_rate; EGRVlv_rOfsLrnVlv input; EGRVlv_rEGR input; EGRVlv_rOfsLrnVlvUnLim output Prc_100_rate; EGRVlv_rAdapIniOpn_C input; EGRVlv_rAdapIniOpn0_C input; EGRVlv_facAdapClsStrt_C input; EGRVlv_rOfsLrnRmpUpFst_C input; EGRVlv_rOfsLrnRmpDwnCls_C input; EGRVlv_ctAdapCls_mp input; EGRVlv_swtEGRTyp2 input; EGRVlv_stTrg_mp input; EGRVlv_swtEGRTyp2T input; EGRVlv_rOfsLrnDwn_C input; EGRVlv_rRmpDwnCls_C input; EGRVlv_rRmpUpFst_C input; EGRVlv_tiStable_C input; EGRVlv_stAdapFin output boolean; EGRVlv_stAdapVlv_mp output boolean; EGRVlv_bEGRVlvOfsLrnJamVlv_DSM output boolean; EGRVlv_stLgTDrft output boolean; EGRVlv_stShTDrft output boolean; EGRVlv_stOfsLrn output State_uint8; EGRVlv_stStr_mp output boolean; EGRVlv_stIntegRmpDwnCls_mp local boolean; EGRVlv_stIntegRmpUpFst_mp local boolean; DT input; EGRVlv_rActUnCor input; EGRVlv_rAdapDiffPlausLgT_C input; EGRVlv_rAdapDiffPlausShT_C input; EGRVlv_rAdapPosAvg_mp input; EGRVlv_rOfsLrnFrst_MR input Prc_100_rate; EGRVlv_rOfsLrnLst_MR input Prc_100_rate; EGRVlv_stOfsLrnFrst input; EGRVlv_tiAdapWaitSensAcq_C input; EGRVlv_bEGRVlvLgTDrft_DSM output boolean; EGRVlv_bEGRVlvShTDrft_DSM output boolean; EGRVlv_rAdapPos_mp output Prc_100_rate; EGRVlv_rOfsLrnFrst_MW output Prc_100_rate; EGRVlv_rOfsLrnLst_MW output Prc_100_rate; EGRVlv_tiStable_mp output Debounce_ms; EGRVlv_tiAdapWaitSensAcq_mp output Debounce_ms; EGRVlv_stWaitElaps local boolean; EGRVlv_stAdpSccs input; EGRVlv_stEdgOpn_mp input; EGRVlv_stFrstOpn_mp input; EGRVlv_stMovFin_mp input; EGRVlv_stPlaus input; EGRVlv_stVlvClsd_mp input; EGRVlv_stVlvStkCls_mp input; EGRVlv_stVlvStk_mp input
  events: Init output FUNCTION_CALL_EVENT; Open output FUNCTION_CALL_EVENT; Close output FUNCTION_CALL_EVENT; Store output FUNCTION_CALL_EVENT; Plausible output FUNCTION_CALL_EVENT
